simulink model "SF004B_AssiSumLim"  (R2013b)
settings: Solver=FixedStepDiscrete  StartTime=0.0  StopTime=1  FixedStep=.002  RelTol=1e-3
values from neighbouring files (symbols this model uses):
  AssiSumLimNtc0x0C4FailStep = DataDict.Calibration    [SF004B_AssiSumLim_DataDict.m]
  AssiSumLimNtc0x0C4PassStep = DataDict.Calibration    [SF004B_AssiSumLim_DataDict.m]
  AssiSumLimPullCmpLim = DataDict.Calibration    [SF004B_AssiSumLim_DataDict.m]
  CMDTHD_MOTNWTMTR_F32 = DataDict.Constant    [SF004B_AssiSumLim_DataDict.m]
  E_NOT_OK = DataDict.Constant    [AR200A_ArSuprt_DataDict.m]
  E_OK = DataDict.Constant    [AR200A_ArSuprt_DataDict.m]
  MOTTQZERO_MOTNWTMTR_F32 = DataDict.Constant    [SF004B_AssiSumLim_DataDict.m]
  VEHSPDTHD_KPH_F32 = DataDict.Constant    [SF004B_AssiSumLim_DataDict.m]
undefined symbols (not defined in the file or in its folder): NtcNr1, NtcSts1, SigQlfr1
libraries: simulink x11, NexteerUtilities x7, NxtrSign x1, NxtrAbslt x1
(part 3 of 3)

== system SF004B_AssiSumLim/AssiSumLim/SetManTqCmd/THEN/If Action Subsystem1 ==
  In1 : Inport
  In2 : Inport  Port=2
  In3 : Inport  Port=3
  Action Port : ActionPort  ActionType=else
  CopyRight2 : Subsystem  Description=|  mask(Copyright Information){none=on}
      | Copyright info block.                                               
      |                                                                     
      | Place copyright information at the top of every subsystem in design.
      mask prompts: none "No parameters"
      mask help: Place copyright information at the top of every subsystem in design.
      mask Display:
      | NxtrConf = 'Nexteer Confidential';
      | 
      | sys = bdroot; %handle for the current model ("system")
      | first = get_param(sys,'Created');
      | first = first(end-3:end);  %year is last four digits
      | 
      | last = get_param(sys,'LastModifiedDate');
      | if isempty(last)
      |     last = datestr(now,'yyyy');
      | else
      |     last = last(end-3:end);
      | end
      | 
      | if strcmp(first,last)
      |     fprintf('%s -- Copyright %s Nexteer',NxtrConf,first)
      | else
      |     fprintf('%s -- %s%s- %s Nexteer',NxtrConf,char(169),first,last)
      | end
  Out1 : Outport
  Out2 : Outport  Port=2
  Out3 : Outport  Port=3
  wires:
  In3/1 -> Out3/1
  In2/1 -> Out2/1
  In1/1 -> Out1/1

== system SF004B_AssiSumLim/ISO Fault Debounce/DiagMgr/NTCSTS_PREFAILD/CopyRight2 ==

== system SF004B_AssiSumLim/ISO Fault Debounce/DiagMgr/NTCSTS_PREFAILD/If Action Subsystem ==
  DS : Inport
  Qlf : Inport  Port=2
  Action Port : ActionPort  ActionType=then
  EAo : Outport
  Qlfo : Outport  Port=2
  wires:
  Qlf/1 -> Qlfo/1
  DS/1 -> EAo/1

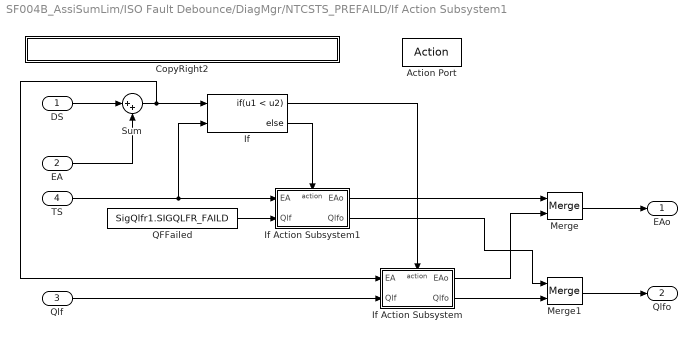
== system SF004B_AssiSumLim/ISO Fault Debounce/DiagMgr/NTCSTS_PREFAILD/If Action Subsystem1 ==
  DS : Inport
  EA : Inport  Port=2
  Qlf : Inport  Port=3
  TS : Inport  Port=4
  Action Port : ActionPort  ActionType=else
  CopyRight2 : Subsystem  Description=|  mask(Copyright Information){none=on}
      | Copyright info block.                                               
      |                                                                     
      | Place copyright information at the top of every subsystem in design.
      mask prompts: none "No parameters"
      mask help: Place copyright information at the top of every subsystem in design.
      mask Display:
      | NxtrConf = 'Nexteer Confidential';
      | 
      | sys = bdroot; %handle for the current model ("system")
      | first = get_param(sys,'Created');
      | first = first(end-3:end);  %year is last four digits
      | 
      | last = get_param(sys,'LastModifiedDate');
      | if isempty(last)
      |     last = datestr(now,'yyyy');
      | else
      |     last = last(end-3:end);
      | end
      | 
      | if strcmp(first,last)
      |     fprintf('%s -- Copyright %s Nexteer',NxtrConf,first)
      | else
      |     fprintf('%s -- %s%s- %s Nexteer',NxtrConf,char(169),first,last)
      | end
  If : If  NumInputs=2  IfExpression=u1 < u2
  If Action Subsystem : Subsystem  TreatAsAtomicUnit=on
  If Action Subsystem1 : Subsystem  TreatAsAtomicUnit=on
  Merge : Merge
  Merge1 : Merge
  QFFailed : Constant  Value=SigQlfr1.SIGQLFR_FAILD  OutDataTypeStr=Enum: SigQlfr1
  Sum : Sum  Inputs=|++
  EAo : Outport
  Qlfo : Outport  Port=2
  wires:
  DS/1 -> Sum/1
  EA/1 -> Sum/2
  Sum/1 -> If Action Subsystem/1(EA), If/1
  TS/1 -> If Action Subsystem1/1(EA), If/2
  If/2 -> If Action Subsystem1/Action
  If/1 -> If Action Subsystem/Action
  Qlf/1 -> If Action Subsystem/2(Qlf)
  QFFailed/1 -> If Action Subsystem1/2(Qlf)
  Merge1/1 -> Qlfo/1
  Merge/1 -> EAo/1
  If Action Subsystem1/1(EAo) -> Merge/1
  If Action Subsystem/1(EAo) -> Merge/2
  If Action Subsystem1/2(Qlfo) -> Merge1/1
  If Action Subsystem/2(Qlfo) -> Merge1/2

== system SF004B_AssiSumLim/ISO Fault Debounce/DiagMgr/NTCSTS_PREPASSD/CopyRight2 ==

== system SF004B_AssiSumLim/ISO Fault Debounce/DiagMgr/NTCSTS_PREPASSD/If Action Subsystem ==
  In1 : Inport
  In2 : Inport  Port=2
  Action Port : ActionPort  ActionType=then
  Out1 : Outport
  Out2 : Outport  Port=2
  wires:
  In1/1 -> Out1/1
  In2/1 -> Out2/1

== system SF004B_AssiSumLim/ISO Fault Debounce/DiagMgr/NTCSTS_PREPASSD/If Action Subsystem1 ==
  In1 : Inport
  In2 : Inport  Port=2
  Action Port : ActionPort  ActionType=else
  Out1 : Outport
  Out2 : Outport  Port=2
  wires:
  In1/1 -> Out1/1
  In2/1 -> Out2/1

== system SF004B_AssiSumLim/AssiSumLim/AssiSumLmtPer1/Safety Check/GetNtcQlfrSts/CopyRight2 ==

== system SF004B_AssiSumLim/AssiSumLim/AssiSumLmtPer1/Safety Check/OK/CopyRight2 ==

== system SF004B_AssiSumLim/AssiSumLim/AssiSumLmtPer1/Safety Check/OK/SetNtcSts ==
  NtcNr : Inport
  NtcStInfo : Inport  Port=2
  NtcSts : Inport  Port=3
  DebStep : Inport  Port=4
  CopyRight2 : Subsystem  Description=|  mask(Copyright Information){none=on}
      | Copyright info block.                                               
      |                                                                     
      | Place copyright information at the top of every subsystem in design.
      mask prompts: none "No parameters"
      mask help: Place copyright information at the top of every subsystem in design.
      mask Display:
      | NxtrConf = 'Nexteer Confidential';
      | 
      | sys = bdroot; %handle for the current model ("system")
      | first = get_param(sys,'Created');
      | first = first(end-3:end);  %year is last four digits
      | 
      | last = get_param(sys,'LastModifiedDate');
      | if isempty(last)
      |     last = datestr(now,'yyyy');
      | else
      |     last = last(end-3:end);
      | end
      | 
      | if strcmp(first,last)
      |     fprintf('%s -- Copyright %s Nexteer',NxtrConf,first)
      | else
      |     fprintf('%s -- %s%s- %s Nexteer',NxtrConf,char(169),first,last)
      | end
  Data Store Write1 : DataStoreWrite  DataStoreName=DebStep
  Data Store Write2 : DataStoreWrite  DataStoreName=NtcSts
  Terminator1 : Terminator
  Terminator2 : Terminator
  wires:
  NtcNr/1 -> Terminator1/1
  NtcSts/1 -> Data Store Write2/1
  DebStep/1 -> Data Store Write1/1
  NtcStInfo/1 -> Terminator2/1

== system SF004B_AssiSumLim/AssiSumLim/AssiSumLmtPer1/Safety Check/Override/CopyRight2 ==

== system SF004B_AssiSumLim/AssiSumLim/AssiSumLmtPer1/Safety Check/Override/SetNtcSts1 ==
  NtcNr : Inport
  NtcStInfo : Inport  Port=2
  NtcSts : Inport  Port=3
  DebStep : Inport  Port=4
  CallDiagMgr : ActionPort  ActionType=then
  Data Store Write1 : DataStoreWrite  DataStoreName=DebStep
  Data Store Write2 : DataStoreWrite  DataStoreName=NtcSts
  Terminator1 : Terminator
  Terminator2 : Terminator
  wires:
  NtcNr/1 -> Terminator1/1
  NtcSts/1 -> Data Store Write2/1
  DebStep/1 -> Data Store Write1/1
  NtcStInfo/1 -> Terminator2/1

== system SF004B_AssiSumLim/AssiSumLim/AssiSumLmtPer1/Safety Check/Override/SetNtcSts2 ==
  NtcNr : Inport
  NtcStInfo : Inport  Port=2
  NtcSts : Inport  Port=3
  DebStep : Inport  Port=4
  CallDiagMgr : ActionPort  ActionType=else
  Data Store Write1 : DataStoreWrite  DataStoreName=DebStep
  Data Store Write2 : DataStoreWrite  DataStoreName=NtcSts
  Terminator : Terminator
  Terminator1 : Terminator
  wires:
  NtcStInfo/1 -> Terminator1/1
  DebStep/1 -> Data Store Write1/1
  NtcSts/1 -> Data Store Write2/1
  NtcNr/1 -> Terminator/1

== system SF004B_AssiSumLim/AssiSumLim/SetManTqCmd/THEN/If Action Subsystem/CopyRight2 ==

== system SF004B_AssiSumLim/AssiSumLim/SetManTqCmd/THEN/If Action Subsystem1/CopyRight2 ==

== system SF004B_AssiSumLim/ISO Fault Debounce/DiagMgr/NTCSTS_PREFAILD/If Action Subsystem1/CopyRight2 ==

== system SF004B_AssiSumLim/ISO Fault Debounce/DiagMgr/NTCSTS_PREFAILD/If Action Subsystem1/If Action Subsystem ==
  EA : Inport
  Qlf : Inport  Port=2
  Action Port : ActionPort  ActionType=then
  EAo : Outport
  Qlfo : Outport  Port=2
  wires:
  EA/1 -> EAo/1
  Qlf/1 -> Qlfo/1

== system SF004B_AssiSumLim/ISO Fault Debounce/DiagMgr/NTCSTS_PREFAILD/If Action Subsystem1/If Action Subsystem1 ==
  EA : Inport
  Qlf : Inport  Port=2
  Action Port : ActionPort  ActionType=else
  EAo : Outport
  Qlfo : Outport  Port=2
  wires:
  EA/1 -> EAo/1
  Qlf/1 -> Qlfo/1

== system SF004B_AssiSumLim/AssiSumLim/AssiSumLmtPer1/Safety Check/OK/SetNtcSts/CopyRight2 ==
